simulink model "BaseMotorSimulink"  (R2020b)
settings: Solver=VariableStepAuto  StartTime=0.0  StopTime=SimTime  FixedStep=solverTimeStep  RelTol=1e-3
InitFcn:
  | StartupScript
undefined symbols (not defined in the file): CF, GearRatiob, Isat, Kb, Kdb, Kib, Kmb, Kpb, PidLim, PidUCGain, r2d, sensorGain, Vsat
libraries: cstblocks x4
settings Model: Creator=nisch  LastModifiedBy=nisch

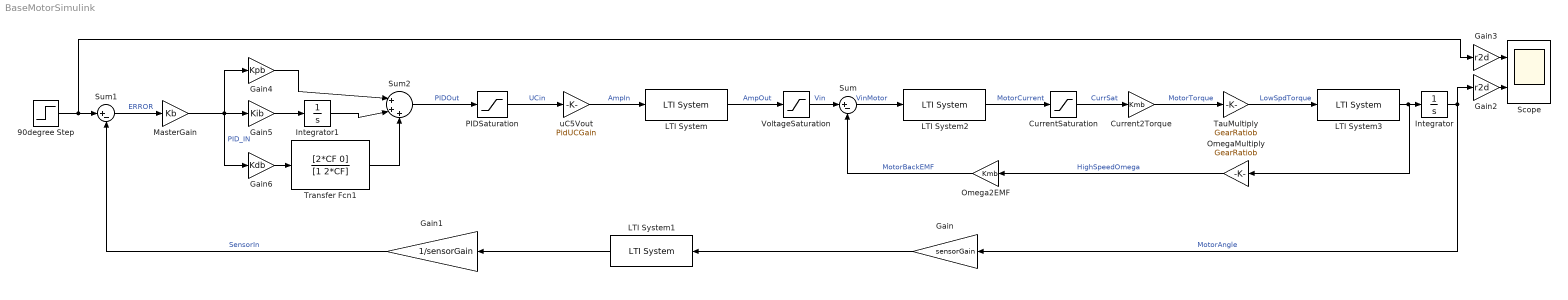
== system BaseMotorSimulink ==
  90degree Step : Step  Time=0  After=pi  SampleTime=0
  Current2Torque : Gain  Gain=Kmb
  CurrentSaturation : Saturate  UpperLimit=Isat  LowerLimit=-Isat
  Gain : Gain  Gain=sensorGain
  Gain1 : Gain  Gain=1/sensorGain
  Gain2 : Gain  Gain=r2d
  Gain3 : Gain  Gain=r2d
  Gain4 : Gain  Gain=Kpb
  Gain5 : Gain  Gain=Kib
  Gain6 : Gain  Gain=Kdb
  Integrator : Integrator
  Integrator1 : Integrator
  LTI System : cstblocks/LTI System  sys=VoltageAmplifier  IC=[]
  LTI System1 : cstblocks/LTI System  sys=Hs  IC=[]
  LTI System2 : cstblocks/LTI System  sys=Electricalb  IC=[]
  LTI System3 : cstblocks/LTI System  sys=Mechanicalb  IC=[]
  MasterGain : Gain  Gain=Kb
  Omega2EMF : Gain  Gain=Kmb
  OmegaMultiply : Gain  Gain=GearRatiob
  PIDSaturation : Saturate  UpperLimit=PidLim  LowerLimit=-PidLim
  Scope : Scope  NumInputPorts=2
  Sum : Sum  Inputs=|+-
  Sum1 : Sum  Inputs=|+-
  Sum2 : Sum  Inputs=|+++
  TauMultiply : Gain  Gain=GearRatiob
  Transfer Fcn1 : TransferFcn  Numerator=[2*CF 0]  Denominator=[1 2*CF]
  VoltageSaturation : Saturate  UpperLimit=Vsat  LowerLimit=-Vsat
  uC5Vout : Gain  Gain=PidUCGain
  wires:
  Sum/1 -> LTI System2/1  "VinMotor"
  Omega2EMF/1 -> Sum/2  "MotorBackEMF"
  LTI System3/1 -> OmegaMultiply/1, Integrator/1
  Sum1/1 -> MasterGain/1  "ERROR"
  Integrator/1 -> Gain2/1, Gain/1  "MotorAngle"
  Gain/1 -> LTI System1/1
  LTI System1/1 -> Gain1/1
  Gain1/1 -> Sum1/2  "SensorIn"
  Gain2/1 -> Scope/2
  Gain3/1 -> Scope/1
  VoltageSaturation/1 -> Sum/1  "Vin"
  MasterGain/1 -> Gain6/1, Gain5/1, Gain4/1  "PID_IN"
  Gain5/1 -> Integrator1/1
  Gain6/1 -> Transfer Fcn1/1
  Sum2/1 -> PIDSaturation/1  "PIDOut"
  Gain4/1 -> Sum2/1
  Integrator1/1 -> Sum2/2
  Transfer Fcn1/1 -> Sum2/3
  LTI System2/1 -> CurrentSaturation/1  "MotorCurrent"
  CurrentSaturation/1 -> Current2Torque/1  "CurrSat"
  Current2Torque/1 -> TauMultiply/1  "MotorTorque"
  TauMultiply/1 -> LTI System3/1  "LowSpdTorque"
  OmegaMultiply/1 -> Omega2EMF/1  "HighSpeedOmega"
  90degree Step/1 -> Gain3/1, Sum1/1
  LTI System/1 -> VoltageSaturation/1  "AmpOut"
  PIDSaturation/1 -> uC5Vout/1  "UCin"
  uC5Vout/1 -> LTI System/1  "AmpIn"
